simulink model "Model1"  (R2020a)
settings: Solver=VariableStepAuto  StartTime=0.0  StopTime=10.0  RelTol=1e-3
model workspace (MAT data in the model file):
  B = 50
  K1 = 50
  K12 = 72.7941176471
  M1 = 100
  M2 = 63.1893382353
settings Model: Creator=HP  LastModifiedBy=HP

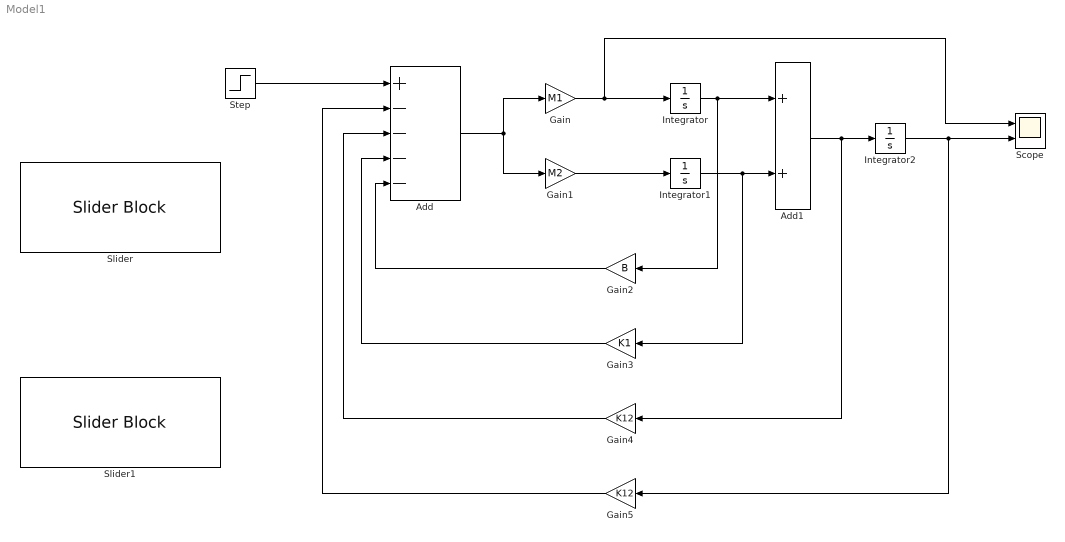
== system Model1 ==
  Add : Sum  Inputs=+----
  Add1 : Sum
  Gain : Gain  Gain=M1
  Gain1 : Gain  Gain=M2
  Gain2 : Gain  Gain=B
  Gain3 : Gain  Gain=K1
  Gain4 : Gain  Gain=K12
  Gain5 : Gain  Gain=K12
  Integrator : Integrator
  Integrator1 : Integrator
  Integrator2 : Integrator
  Scope : Scope  NumInputPorts=2
  Slider : SliderBlock
  Slider1 : SliderBlock
  Step : Step  SampleTime=0
  wires:
  Gain2/1 -> Add/5
  Gain3/1 -> Add/4
  Gain4/1 -> Add/3
  Gain5/1 -> Add/2
  Integrator/1 -> Add1/1, Gain2/1
  Integrator1/1 -> Add1/2, Gain3/1
  Add1/1 -> Integrator2/1, Gain4/1
  Integrator2/1 -> Gain5/1, Scope/2
  Add/1 -> Gain1/1, Gain/1
  Gain/1 -> Scope/1, Integrator/1
  Gain1/1 -> Integrator1/1
  Step/1 -> Add/1
